simulink model "motor_curent_continuu"  (R2024a)
settings: Solver=VariableStepAuto  StartTime=0.0  StopTime=50  RelTol=1e-3
values from neighbouring files (symbols this model uses):
  A = [-1/Ta -ke/La; km/J 0]    [parametri.m]
  B = [kE/La 0; 0 -1/J]    [parametri.m]
  C = eye(2)    [parametri.m]
  D = zeros(2)    [parametri.m]
  J = 0.0302    [parametri.m]
  kE = 42.85    [parametri.m]
  ke = 0.56    [parametri.m]
  km = 0.55    [parametri.m]
  Ra = 5.1    [parametri.m]
  Ta = 0.1    [parametri.m]
  Tm = 0.5    [parametri.m]
settings Model: Creator=paulhondola  LastModifiedBy=paulhondola

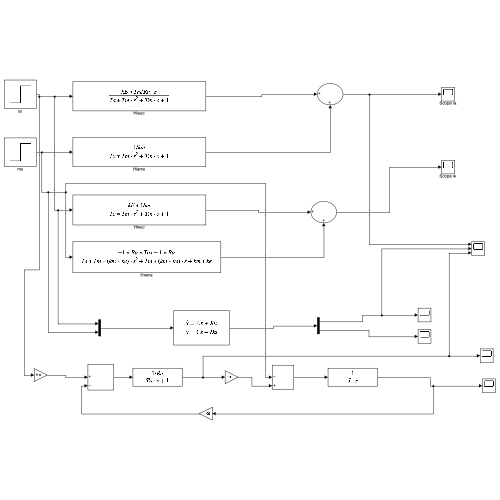
[thumbnail: Simulink's stored preview of the top-level diagram]
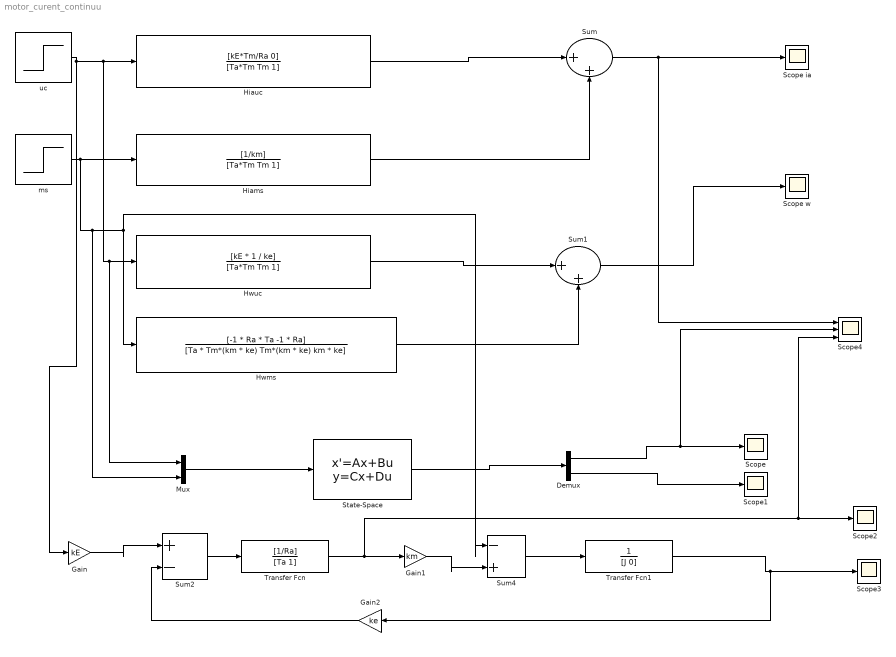
== system motor_curent_continuu ==
  Demux : Demux  Outputs=2
  Gain : Gain  Gain=kE
  Gain1 : Gain  Gain=km
  Gain2 : Gain  Gain=ke
  Hiams : TransferFcn  Numerator=[1/km]  Denominator=[Ta*Tm Tm 1]
  Hiauc : TransferFcn  Numerator=[kE*Tm/Ra 0]  Denominator=[Ta*Tm Tm 1]
  Hwms : TransferFcn  Numerator=[-1 * Ra * Ta -1 * Ra]  Denominator=[Ta * Tm*(km * ke) Tm*(km * ke) km * ke]
  Hwuc : TransferFcn  Numerator=[kE * 1 / ke]  Denominator=[Ta*Tm Tm 1]
  Mux : Mux  Inputs=2
  Scope{,1..3} (4 alike) : Scope
  Scope ia : Scope
  Scope w : Scope
  Scope4 : Scope  NumInputPorts=3
  State-Space : StateSpace  A=A  B=B  C=C  D=D  InitialCondition=0
  Sum : Sum  Inputs=|++
  Sum1 : Sum  Inputs=|++
  Sum2 : Sum  Inputs=|+-
  Sum4 : Sum  Inputs=|-+
  Transfer Fcn : TransferFcn  Numerator=[1/Ra]  Denominator=[Ta 1]
  Transfer Fcn1 : TransferFcn  Denominator=[J 0]
  ms : Step  Time=30  SampleTime=0
  uc : Step  Time=0  After=3.5  SampleTime=0
  wires:
  Hiauc/1 -> Sum/1
  Hiams/1 -> Sum/2
  Sum/1 -> Scope4/1, Scope ia/1
  Hwuc/1 -> Sum1/1
  Hwms/1 -> Sum1/2
  Sum1/1 -> Scope w/1
  Mux/1 -> State-Space/1
  State-Space/1 -> Demux/1
  Demux/1 -> Scope4/2, Scope/1
  Demux/2 -> Scope1/1
  Gain/1 -> Sum2/1
  Gain1/1 -> Sum4/2
  ms/1 -> Mux/2, Sum4/1, Hwms/1, Hiams/1
  uc/1 -> Mux/1, Hwuc/1, Hiauc/1, Gain/1
  Sum4/1 -> Transfer Fcn1/1
  Gain2/1 -> Sum2/2
  Sum2/1 -> Transfer Fcn/1
  Transfer Fcn/1 -> Scope4/3, Scope2/1, Gain1/1
  Transfer Fcn1/1 -> Gain2/1, Scope3/1
